simulink model "Pid"  (R2023b)
settings: Solver=ode4  StartTime=0.0  StopTime=1000  FixedStep=0.1  RelTol=1e-3
values from neighbouring files (symbols this model uses):
  k = 0.036    [date_personalizate.m]    (also in grafice.m = 0.035)
  k11 = k2^2+4*(k-k3)*k1    (= 0.0915786)    [date_personalizate.m]
  k12 = 8*(k-k3)    (= 0.2928)    [date_personalizate.m]
  k13 = 2*(k-k3)    (= 0.0732)    [date_personalizate.m]
  k2 = -0.015    [date_personalizate.m]    (also in grafice.m)
  keta = 8e-5    (= 8e-05)    [date_personalizate.m]
libraries: instrumentlib x2
settings Model: Creator=40787  LastModifiedBy=40787

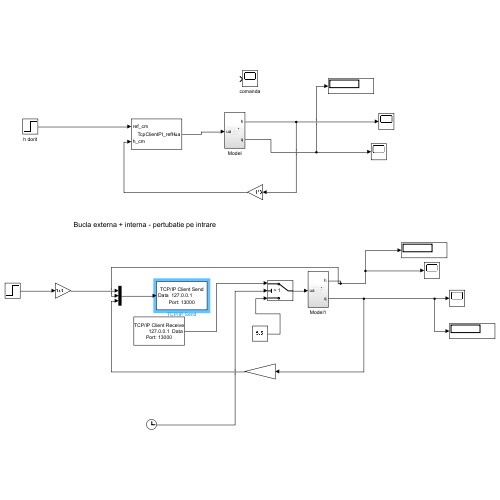
[thumbnail: Simulink's stored preview of the top-level diagram]
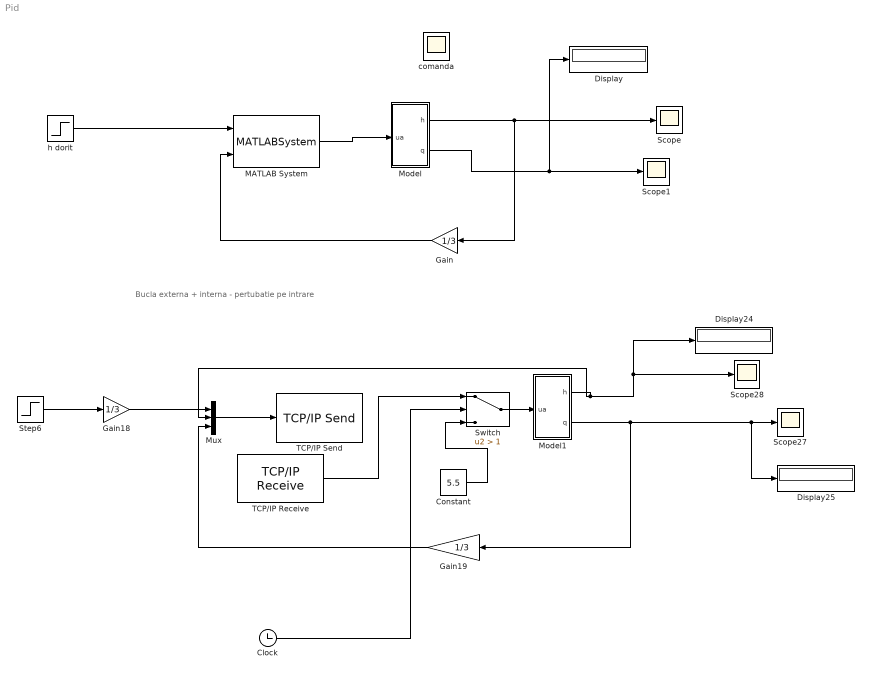
== system Pid ==
  note: Bucla externa + interna - pertubatie pe intrare
  Clock : Clock
  Constant : Constant  Value=5.5
  Display : Display
  Display24 : Display
  Display25 : Display
  Gain : Gain  Gain=1/3
  Gain18 : Gain  Gain=1/3
  Gain19 : Gain  Gain=1/3
  MATLAB System : MATLABSystem  System=TcpClientPI_refH  ServerIP=127.0.0.1  ServerPort=25000  Timeout=5  SimulateUsing=Code generation
      mask Type: TcpClientPI_refH
      mask Display:
      | disp('TcpClientPI_refH');
      | port_label('input',1,'ref_cm');
      | port_label('input',2,'h_cm');
      | port_label('output',1,'ua');
  Model : Subsystem
  Model1 : Subsystem
  Mux : Mux  Inputs=3
  Scope{,1,27..28} (4 alike) : Scope
  Step6 : Step  After=20  SampleTime=0
  Switch : Switch  Criteria=u2 > Threshold  Threshold=1  SaturateOnIntegerOverflow=off  InputSameDT=off
  TCP/IP Receive : instrumentlib/TCP//IP Receive  Host=127.0.0.1  Port=13000  DataSize=1  DataType=double  ASCIIFormatting=%f  Terminator=LF  CustomTerminator=10  ByteOrder=little-endian  EnableBlockingMode=on  Timeout=20  SampleTime=0.1  SimulateUsing=Interpreted execution
  TCP/IP Send : instrumentlib/TCP//IP Send  Host=127.0.0.1  Port=13000  ByteOrder=little-endian  EnableBlockingMode=on  Timeout=10  TransferDelay=on  SimulateUsing=Interpreted execution
  comanda : Scope
  h dorit : Step  Time=0  After=13  SampleTime=0
  wires:
  Model/1(h) -> Gain/1, Scope/1
  Model/2(q) -> Scope1/1, Display/1
  Gain/1 -> MATLAB System/2
  h dorit/1 -> MATLAB System/1
  MATLAB System/1 -> Model/1(ua)
  Switch/1 -> Model1/1(ua)
  Constant/1 -> Switch/3
  TCP/IP Receive/1 -> Switch/1
  Clock/1 -> Switch/2
  Model1/1(h) -> Mux/2, Display24/1, Scope28/1
  Mux/1 -> TCP/IP Send/1
  Model1/2(q) -> Gain19/1, Display25/1, Scope27/1
  Gain19/1 -> Mux/3
  Gain18/1 -> Mux/1
  Step6/1 -> Gain18/1

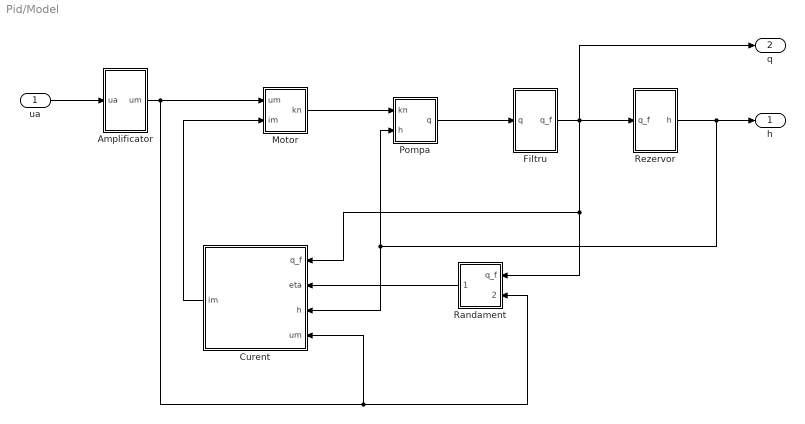
== system Pid/Model ==
  ua : Inport
  "Amplificator " : Subsystem
  Curent : Subsystem
  Filtru : Subsystem
  Motor : Subsystem
  Pompa : Subsystem
  Randament : Subsystem
  Rezervor : Subsystem
  h : Outport
  q : Outport  Port=2
  wires:
  ua/1 -> "Amplificator "/1(ua)
  Motor/1(kn) -> Pompa/1(kn)
  "Amplificator "/1(um) -> Curent/4(um), Randament/2(um), Motor/1(um)
  Rezervor/1(h) -> h/1, Curent/3(h), Pompa/2(h)
  Curent/1(im) -> Motor/2(im)
  Filtru/1(q_f) -> q/1, Rezervor/1(q_f), Curent/1(q_f), Randament/1(q_f)
  Randament/1(eta) -> Curent/2(eta)
  Pompa/1(q) -> Filtru/1(q)

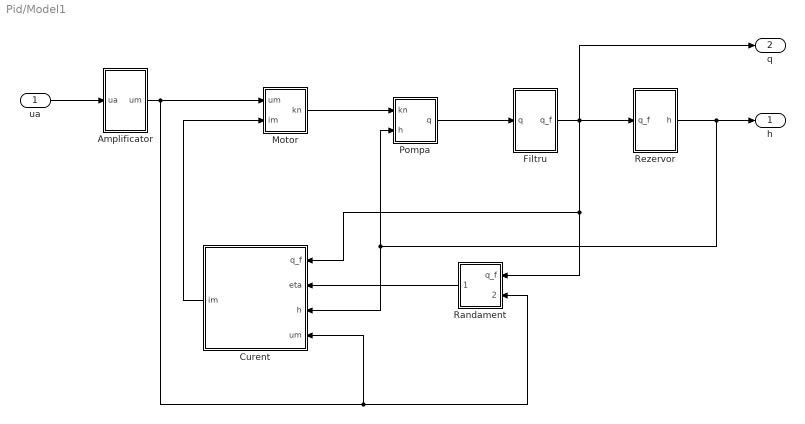
== system Pid/Model1 ==
  ua : Inport
  "Amplificator " : Subsystem
  Curent : Subsystem
  Filtru : Subsystem
  Motor : Subsystem
  Pompa : Subsystem
  Randament : Subsystem
  Rezervor : Subsystem
  h : Outport
  q : Outport  Port=2
  wires:
  ua/1 -> "Amplificator "/1(ua)
  Motor/1(kn) -> Pompa/1(kn)
  "Amplificator "/1(um) -> Curent/4(um), Randament/2(um), Motor/1(um)
  Rezervor/1(h) -> h/1, Curent/3(h), Pompa/2(h)
  Curent/1(im) -> Motor/2(im)
  Filtru/1(q_f) -> q/1, Rezervor/1(q_f), Curent/1(q_f), Randament/1(q_f)
  Randament/1(eta) -> Curent/2(eta)
  Pompa/1(q) -> Filtru/1(q)

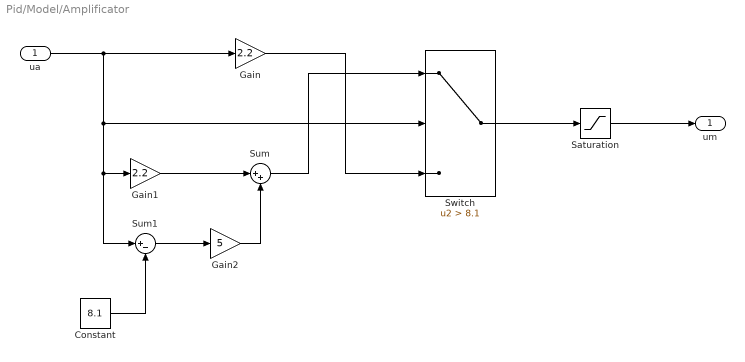
== system Pid/Model/Amplificator  ==
  ua : Inport
  Constant : Constant  Value=8.1
  Gain : Gain  Gain=2.2
  Gain1 : Gain  Gain=2.2
  Gain2 : Gain  Gain=5
  Saturation : Saturate  UpperLimit=22  LowerLimit=0
  Sum : Sum  Inputs=|++
  Sum1 : Sum  Inputs=|+-
  Switch : Switch  Criteria=u2 > Threshold  Threshold=8.1  SaturateOnIntegerOverflow=off  InputSameDT=off
  um : Outport
  wires:
  Gain2/1 -> Sum/2
  Gain1/1 -> Sum/1
  Sum1/1 -> Gain2/1
  Sum/1 -> Switch/1
  ua/1 -> Gain/1, Gain1/1, Sum1/1, Switch/2
  Constant/1 -> Sum1/2
  Gain/1 -> Switch/3
  Switch/1 -> Saturation/1
  Saturation/1 -> um/1

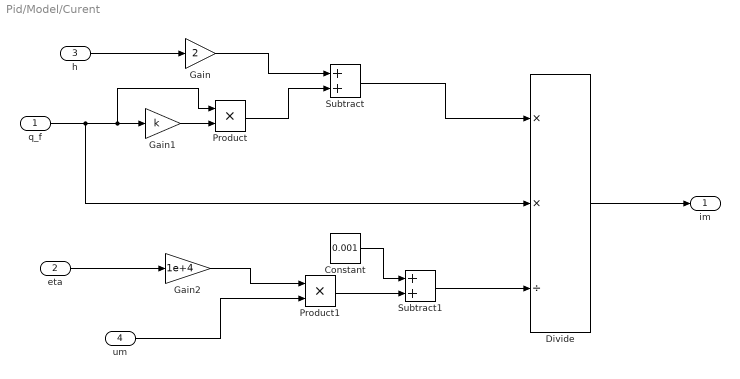
== system Pid/Model/Curent ==
  q_f : Inport
  eta : Inport  Port=2
  h : Inport  Port=3
  um : Inport  Port=4
  Constant : Constant  Value=0.001
  Divide : Product  Inputs=**/
  Gain : Gain  Gain=2
  Gain1 : Gain  Gain=k
  Gain2 : Gain  Gain=1e+4
  Product : Product
  Product1 : Product
  Subtract : Sum
  Subtract1 : Sum
  im : Outport
  wires:
  um/1 -> Product1/2
  h/1 -> Gain/1
  Product1/1 -> Subtract1/2
  eta/1 -> Gain2/1
  Gain/1 -> Subtract/1
  Constant/1 -> Subtract1/1
  Subtract/1 -> Divide/1
  Gain2/1 -> Product1/1
  Product/1 -> Subtract/2
  Subtract1/1 -> Divide/3
  q_f/1 -> Product/1, Gain1/1, Divide/2
  Divide/1 -> im/1
  Gain1/1 -> Product/2

== system Pid/Model/Filtru ==
  q : Inport
  Integrator1 : Integrator  InitialCondition=29.18
  Sum1 : Sum  Inputs=|+-
  q_f : Outport
  wires:
  Sum1/1 -> Integrator1/1
  Integrator1/1 -> q_f/1, Sum1/2
  q/1 -> Sum1/1

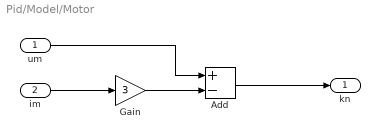
== system Pid/Model/Motor ==
  um : Inport
  im : Inport  Port=2
  Add : Sum  Inputs=+-
  Gain : Gain  Gain=3
  kn : Outport
  wires:
  Gain/1 -> Add/2
  im/1 -> Gain/1
  um/1 -> Add/1
  Add/1 -> kn/1

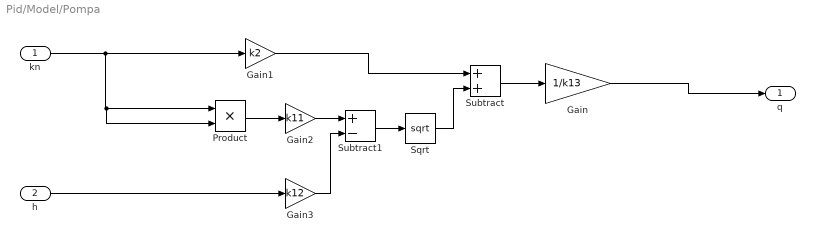
== system Pid/Model/Pompa ==
  kn : Inport
  h : Inport  Port=2
  Gain : Gain  Gain=1/k13
  Gain1 : Gain  Gain=k2
  Gain2 : Gain  Gain=k11
  Gain3 : Gain  Gain=k12
  Product : Product
  Sqrt : Sqrt
  Subtract : Sum
  Subtract1 : Sum  Inputs=+-
  q : Outport
  wires:
  Subtract/1 -> Gain/1
  Sqrt/1 -> Subtract/2
  kn/1 -> Product/2, Product/1, Gain1/1
  Gain3/1 -> Subtract1/2
  Subtract1/1 -> Sqrt/1
  Gain1/1 -> Subtract/1
  h/1 -> Gain3/1
  Product/1 -> Gain2/1
  Gain2/1 -> Subtract1/1
  Gain/1 -> q/1

== system Pid/Model/Randament ==
  q_f : Inport
  um : Inport  Port=2
  Gain : Gain  Gain=keta
  Product : Product
  eta : Outport
  wires:
  Gain/1 -> Product/2
  um/1 -> Gain/1
  q_f/1 -> Product/1
  Product/1 -> eta/1

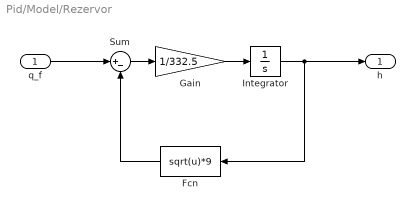
== system Pid/Model/Rezervor ==
  q_f : Inport
  Fcn : Fcn  Expr=sqrt(u)*9
  Gain : Gain  Gain=1/332.5
  Integrator : Integrator  InitialCondition=10.51
  Sum : Sum  Inputs=|+-
  h : Outport
  wires:
  Gain/1 -> Integrator/1
  q_f/1 -> Sum/1
  Integrator/1 -> h/1, Fcn/1
  Sum/1 -> Gain/1
  Fcn/1 -> Sum/2

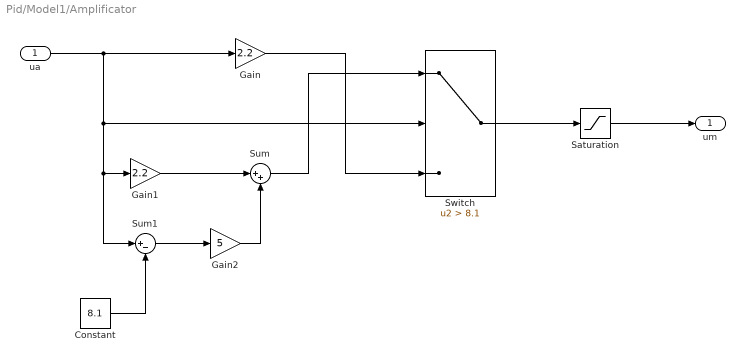
== system Pid/Model1/Amplificator  ==
  ua : Inport
  Constant : Constant  Value=8.1
  Gain : Gain  Gain=2.2
  Gain1 : Gain  Gain=2.2
  Gain2 : Gain  Gain=5
  Saturation : Saturate  UpperLimit=22  LowerLimit=0
  Sum : Sum  Inputs=|++
  Sum1 : Sum  Inputs=|+-
  Switch : Switch  Criteria=u2 > Threshold  Threshold=8.1  SaturateOnIntegerOverflow=off  InputSameDT=off
  um : Outport
  wires:
  Gain2/1 -> Sum/2
  Gain1/1 -> Sum/1
  Sum1/1 -> Gain2/1
  Sum/1 -> Switch/1
  ua/1 -> Gain/1, Gain1/1, Sum1/1, Switch/2
  Constant/1 -> Sum1/2
  Gain/1 -> Switch/3
  Switch/1 -> Saturation/1
  Saturation/1 -> um/1

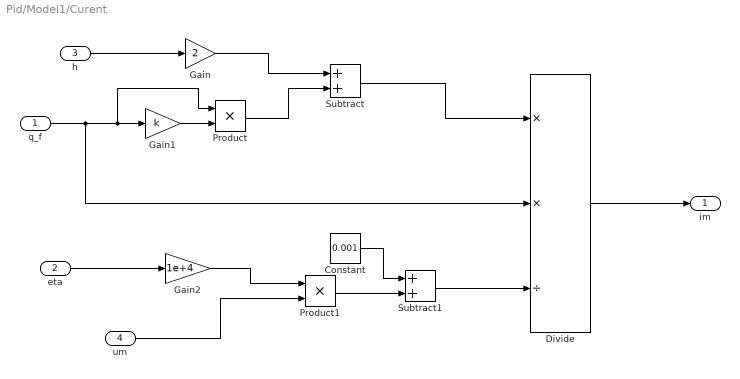
== system Pid/Model1/Curent ==
  q_f : Inport
  eta : Inport  Port=2
  h : Inport  Port=3
  um : Inport  Port=4
  Constant : Constant  Value=0.001
  Divide : Product  Inputs=**/
  Gain : Gain  Gain=2
  Gain1 : Gain  Gain=k
  Gain2 : Gain  Gain=1e+4
  Product : Product
  Product1 : Product
  Subtract : Sum
  Subtract1 : Sum
  im : Outport
  wires:
  um/1 -> Product1/2
  h/1 -> Gain/1
  Product1/1 -> Subtract1/2
  eta/1 -> Gain2/1
  Gain/1 -> Subtract/1
  Constant/1 -> Subtract1/1
  Subtract/1 -> Divide/1
  Gain2/1 -> Product1/1
  Product/1 -> Subtract/2
  Subtract1/1 -> Divide/3
  q_f/1 -> Product/1, Gain1/1, Divide/2
  Divide/1 -> im/1
  Gain1/1 -> Product/2

== system Pid/Model1/Filtru ==
  q : Inport
  Integrator1 : Integrator  InitialCondition=29.18
  Sum1 : Sum  Inputs=|+-
  q_f : Outport
  wires:
  Sum1/1 -> Integrator1/1
  Integrator1/1 -> q_f/1, Sum1/2
  q/1 -> Sum1/1

== system Pid/Model1/Motor ==
  um : Inport
  im : Inport  Port=2
  Add : Sum  Inputs=+-
  Gain : Gain  Gain=3
  kn : Outport
  wires:
  Gain/1 -> Add/2
  im/1 -> Gain/1
  um/1 -> Add/1
  Add/1 -> kn/1

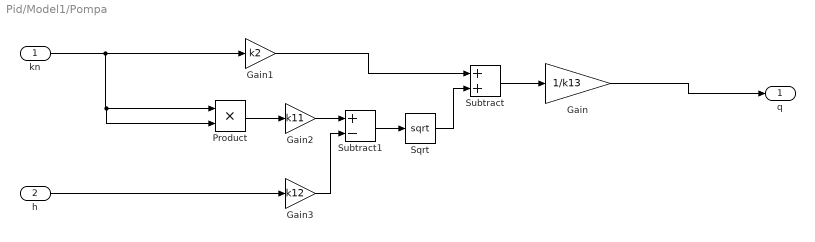
== system Pid/Model1/Pompa ==
  kn : Inport
  h : Inport  Port=2
  Gain : Gain  Gain=1/k13
  Gain1 : Gain  Gain=k2
  Gain2 : Gain  Gain=k11
  Gain3 : Gain  Gain=k12
  Product : Product
  Sqrt : Sqrt
  Subtract : Sum
  Subtract1 : Sum  Inputs=+-
  q : Outport
  wires:
  Subtract/1 -> Gain/1
  Sqrt/1 -> Subtract/2
  kn/1 -> Product/2, Product/1, Gain1/1
  Gain3/1 -> Subtract1/2
  Subtract1/1 -> Sqrt/1
  Gain1/1 -> Subtract/1
  h/1 -> Gain3/1
  Product/1 -> Gain2/1
  Gain2/1 -> Subtract1/1
  Gain/1 -> q/1

== system Pid/Model1/Randament ==
  q_f : Inport
  um : Inport  Port=2
  Gain : Gain  Gain=keta
  Product : Product
  eta : Outport
  wires:
  Gain/1 -> Product/2
  um/1 -> Gain/1
  q_f/1 -> Product/1
  Product/1 -> eta/1

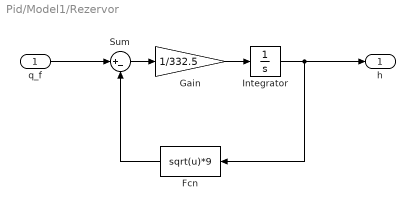
== system Pid/Model1/Rezervor ==
  q_f : Inport
  Fcn : Fcn  Expr=sqrt(u)*9
  Gain : Gain  Gain=1/332.5
  Integrator : Integrator  InitialCondition=10.51
  Sum : Sum  Inputs=|+-
  h : Outport
  wires:
  Gain/1 -> Integrator/1
  q_f/1 -> Sum/1
  Integrator/1 -> h/1, Fcn/1
  Sum/1 -> Gain/1
  Fcn/1 -> Sum/2
